simulink model "vi_sweep_stream_matlab"  (R2025b)
settings: Solver=FixedStepDiscrete  StartTime=0.0  StopTime=inf  FixedStep=1  RelTol=1e-3
settings Model: Creator=nop  LastModifiedBy=nop

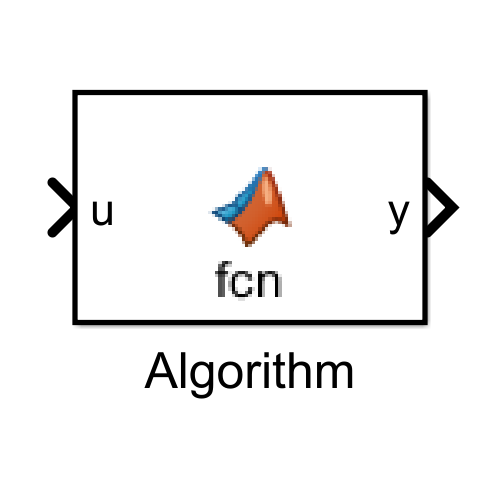
[thumbnail: Simulink's stored preview of the top-level diagram]
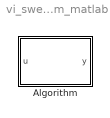
== system vi_sweep_stream_matlab ==
  Algorithm : MATLAB Function  TreatAsAtomicUnit=on

== matlab function vi_sweep_stream_matlab/Algorithm ==
  data: u input; y output
function y = fcn(u)

y = u;
